simulink model "MdXXIsPosChk"  (R2024b)
settings: Solver=FixedStepDiscrete  StartTime=0.0  StopTime=10.0  FixedStep=0.01  RelTol=1e-3
libraries: simulink x35
(part 1 of 2)
settings Model: Creator=sn2xws  LastModifiedBy=sn55gm
settings Model: ModifiedHistory=|
  | 2024.5.6
  | 557 新增零重力电机
  | V3.0.1 2024.7.9 557模式流程V1.9
  | V3.0.2 2024.8.14 修复6slug无法报成功的问题
  | V3.0.3 Md18报成功的逻辑变更
  | V3.0.4 Md29报成功逻辑变更
  | V3.0.5 Md2，Md3，Md29到位置的逻辑更改（BUG924822）
  | V3.0.6 Md2，Md3，Md29到位置的逻辑更改（BUG924822），会默认到位置，需要先把到位置位置0
  | V3.0.7 Md32 只要靠背折叠到位置，modeposalready赋值1
  | V3.0.8 Md12 不看副驾到位
  | V3.0.9 Md30 Md31成功不看副驾前后
  | V3.1.0 Md30 Md31posalready 也不看副驾前后
  | V3.13.0 Md30 Md31成功不看二排腿托和延伸
settings SolverCC: AlgebraicLoopSolver=TrustRegion
settings DataIOCC: SaveFormat=StructureWithTime  ReturnWorkspaceOutputs=off
settings OptimizationCC: DefaultParameterBehavior=Inlined  EnhancedBackFolding=on  PassReuseOutputArgsAs=Individual arguments  ZeroExternalMemoryAtStartup=off  ZeroInternalMemoryAtStartup=off  OptimizeBlockOrder=speed  DifferentSizesBufferReuse=on  OptimizationCustomize=off  EfficientTunableParamExpr=on
settings DebuggingCC: ParameterTunabilityLossMsg=error  UnconnectedInputMsg=warning  UnconnectedOutputMsg=warning  UnconnectedLineMsg=warning  ArithmeticOperatorsInVariantConditions=warning
settings ModelReferenceCC: EnableRefExpFcnMdlSchedulingChecks=on  ModelReferenceNumInstancesAllowed=Single
settings SFSimCC: MATLABDynamicMemAlloc=off  CustomCodeUndefinedFunction=UseInterfaceOnly
settings RTWCC: Description=AUTOSAR  SystemTargetFile=autosar.tlc  GenCodeOnly=on  TemplateMakefile=ert_default_tmf  GenerateReport=on  IncludeHyperlinkInReport=on  LaunchReport=on  DataTypeReplacement=CDataTypesFixedWidth  GenerateTraceInfo=on  GenerateTraceReport=on  GenerateTraceReportSl=on  GenerateTraceReportSf=on  GenerateTraceReportEml=on  GenerateCodeMetricsReport=on  GPUComputeCapability=3.5
settings CodeAppCC: ForceParamTrailComments=on  IgnoreCustomStorageClasses=off  OperatorAnnotations=on  SimulinkDataObjDesc=on  SFDataObjDesc=on  InsertBlockDesc=on
settings STFCustomTargetCC: TargetLangStandard=C99 (ISO)  MultiwordLength=256  ParMdlRefBuildCompliant=on  CompOptLevelCompliant=on  IncludeMdlTerminateFcn=off  CombineOutputUpdateFcns=on  SuppressErrorStatus=on  ERTCustomFileBanners=on  SupportNonFinite=off  SupportComplex=off  SupportContinuousTime=off  SupportNonInlinedSFcns=off  RemoveResetFunc=on  MATLABClassNameForMDSCustomization=Simulink.SoftwareTarget.ERTCustomization  AutosarCompliant=on  UseToolchainInfoCompliant=on  LookupTableObjectStructAxisOrder=2,1,3,4,...  LUTObjectStructOrderEvenSpacing=Size,Table,Breakpoints  SystemTargetFile=autosar.tlc
settings ERTTargetCC: TargetLangStandard=C99 (ISO)  ConcurrentExecutionCompliant=off  IncludeMdlTerminateFcn=off  SuppressErrorStatus=on  SupportNonFinite=off  SupportComplex=off  ModelStepFunctionPrototypeControlCompliant=off  CPPClassGenCompliant=off  AutosarCompliant=on  LookupTableObjectStructAxisOrder=2,1,3,4,...  LUTObjectStructOrderEvenSpacing=Size,Table,Breakpoints  ERTCustomFileTemplate=example_file_process.tlc  ERTFilePackagingFormat=Compact  BooleanTrueId=TRUE  BooleanFalseId=FALSE  DynamicArrayContainerType=coder::array

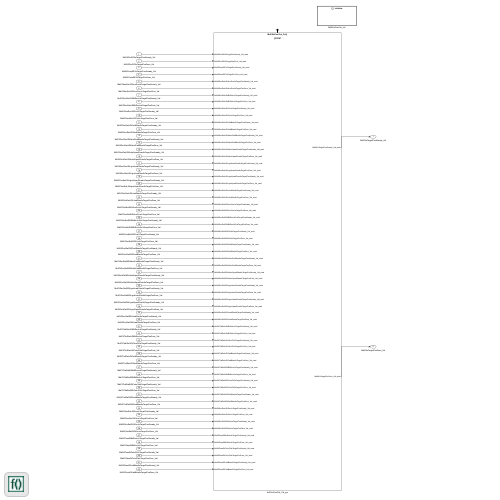
[thumbnail: Simulink's stored preview of the top-level diagram]
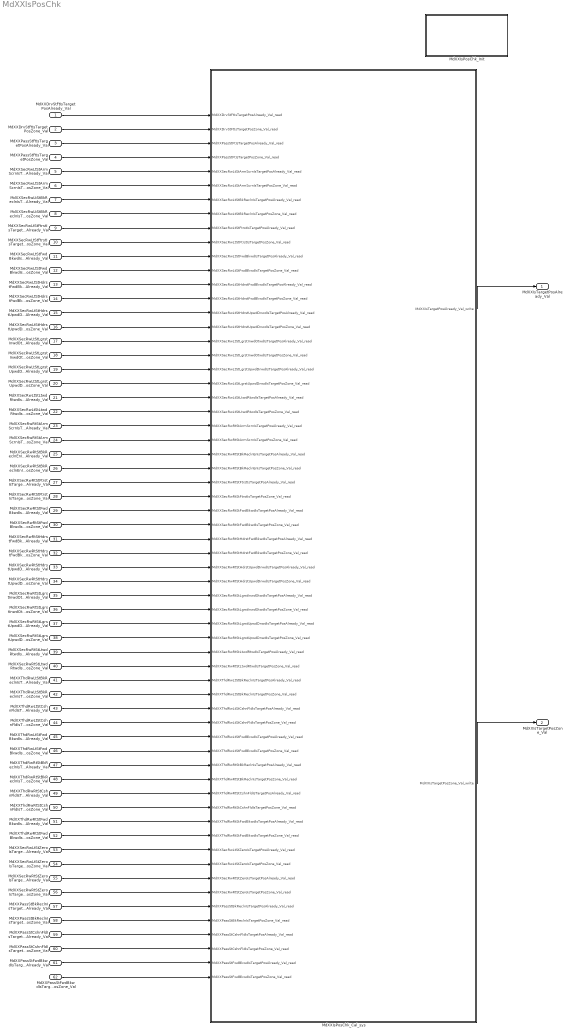
== system MdXXIsPosChk ==
  MdXXDrvStFtIsTargetPosAlready_Val : Inport  OutDataTypeStr=uint32  PortDimensions=1
  MdXXDrvStFtIsTargetPosZone_Val : Inport  Port=2  OutDataTypeStr=uint32  PortDimensions=1
  MdXXPassStFtIsTargetPosAlready_Val : Inport  Port=3  OutDataTypeStr=uint32  PortDimensions=1
  MdXXPassStFtIsTargetPosZone_Val : Inport  Port=4  OutDataTypeStr=uint32  PortDimensions=1
  MdXXSecRwLtStArmScrnIsTargetPosAlready_Val : Inport  Port=5  OutDataTypeStr=uint32  PortDimensions=1
  MdXXSecRwLtStArmScrnIsTargetPosZone_Val : Inport  Port=6  OutDataTypeStr=uint32  PortDimensions=1
  MdXXSecRwLtStBkReclnIsTargetPosAlready_Val : Inport  Port=7  OutDataTypeStr=uint32  PortDimensions=1
  MdXXSecRwLtStBkReclnIsTargetPosZone_Val : Inport  Port=8  OutDataTypeStr=uint32  PortDimensions=1
  MdXXSecRwLtStFtrstIsTargetPosAlready_Val : Inport  Port=9  OutDataTypeStr=uint32  PortDimensions=1
  MdXXSecRwLtStFtrstIsTargetPosZone_Val : Inport  Port=10  OutDataTypeStr=uint32  PortDimensions=1
  MdXXSecRwLtStFwdBkwdIsTargetPosAlready_Val : Inport  Port=11  OutDataTypeStr=uint32  PortDimensions=1
  MdXXSecRwLtStFwdBkwdIsTargetPosZone_Val : Inport  Port=12  OutDataTypeStr=uint32  PortDimensions=1
  MdXXSecRwLtStHdrstFwdBkwdIsTargetPosAlready_Val : Inport  Port=13  OutDataTypeStr=uint32  PortDimensions=1
  MdXXSecRwLtStHdrstFwdBkwdIsTargetPosZone_Val : Inport  Port=14  OutDataTypeStr=uint32  PortDimensions=1
  MdXXSecRwLtStHdrstUpwdDnwdIsTargetPosAlready_Val : Inport  Port=15  OutDataTypeStr=uint32  PortDimensions=1
  MdXXSecRwLtStHdrstUpwdDnwdIsTargetPosZone_Val : Inport  Port=16  OutDataTypeStr=uint32  PortDimensions=1
  MdXXSecRwLtStLgrstInwdOtwdIsTargetPosAlready_Val : Inport  Port=17  OutDataTypeStr=uint32  PortDimensions=1
  MdXXSecRwLtStLgrstInwdOtwdIsTargetPosZone_Val : Inport  Port=18  OutDataTypeStr=uint32  PortDimensions=1
  MdXXSecRwLtStLgrstUpwdDnwdIsTargetPosAlready_Val : Inport  Port=19  OutDataTypeStr=uint32  PortDimensions=1
  MdXXSecRwLtStLgrstUpwdDnwdIsTargetPosZone_Val : Inport  Port=20  OutDataTypeStr=uint32  PortDimensions=1
  MdXXSecRwLtStLtwdRtwdIsTargetPosAlready_Val : Inport  Port=21  OutDataTypeStr=uint32  PortDimensions=1
  MdXXSecRwLtStLtwdRtwdIsTargetPosZone_Val : Inport  Port=22  OutDataTypeStr=uint32  PortDimensions=1
  MdXXSecRwRtStArmScrnIsTargetPosAlready_Val : Inport  Port=23  OutDataTypeStr=uint32  PortDimensions=1
  MdXXSecRwRtStArmScrnIsTargetPosZone_Val : Inport  Port=24  OutDataTypeStr=uint32  PortDimensions=1
  MdXXSecRwRtStBkReclnEnIsTargetPosAlready_Val : Inport  Port=25  OutDataTypeStr=uint32  PortDimensions=1
  MdXXSecRwRtStBkReclnEnIsTargetPosZone_Val : Inport  Port=26  OutDataTypeStr=uint32  PortDimensions=1
  MdXXSecRwRtStFtrstIsTargetPosAlready_Val : Inport  Port=27  OutDataTypeStr=uint32  PortDimensions=1
  MdXXSecRwRtStFtrstIsTargetPosZone_Val : Inport  Port=28  OutDataTypeStr=uint32  PortDimensions=1
  MdXXSecRwRtStFwdBkwdIsTargetPosAlready_Val : Inport  Port=29  OutDataTypeStr=uint32  PortDimensions=1
  MdXXSecRwRtStFwdBkwdIsTargetPosZone_Val : Inport  Port=30  OutDataTypeStr=uint32  PortDimensions=1
  MdXXSecRwRtStHdrstFwdBkwdIsTargetPosAlready_Val : Inport  Port=31  OutDataTypeStr=uint32  PortDimensions=1
  MdXXSecRwRtStHdrstFwdBkwdIsTargetPosZone_Val : Inport  Port=32  OutDataTypeStr=uint32  PortDimensions=1
  MdXXSecRwRtStHdrstUpwdDnwdIsTargetPosAlready_Val : Inport  Port=33  OutDataTypeStr=uint32  PortDimensions=1
  MdXXSecRwRtStHdrstUpwdDnwdIsTargetPosZone_Val : Inport  Port=34  OutDataTypeStr=uint32  PortDimensions=1
  MdXXSecRwRtStLgrstInwdOtwdIsTargetPosAlready_Val : Inport  Port=35  OutDataTypeStr=uint32  PortDimensions=1
  MdXXSecRwRtStLgrstInwdOtwdIsTargetPosZone_Val : Inport  Port=36  OutDataTypeStr=uint32  PortDimensions=1
  MdXXSecRwRtStLgrstUpwdDnwdIsTargetPosAlready_Val : Inport  Port=37  OutDataTypeStr=uint32  PortDimensions=1
  MdXXSecRwRtStLgrstUpwdDnwdIsTargetPosZone_Val : Inport  Port=38  OutDataTypeStr=uint32  PortDimensions=1
  MdXXSecRwRtStLtwdRtwdIsTargetPosAlready_Val : Inport  Port=39  OutDataTypeStr=uint32  PortDimensions=1
  MdXXSecRwRtStLtwdRtwdIsTargetPosZone_Val : Inport  Port=40  OutDataTypeStr=uint32  PortDimensions=1
  MdXXThdRwLtStBkReclnIsTargetPosAlready_Val : Inport  Port=41  OutDataTypeStr=uint32  PortDimensions=1
  MdXXThdRwLtStBkReclnIsTargetPosZone_Val : Inport  Port=42  OutDataTypeStr=uint32  PortDimensions=1
  MdXXThdRwLtStCshnFldIsTargetPosAlready_Val : Inport  Port=43  OutDataTypeStr=uint32  PortDimensions=1
  MdXXThdRwLtStCshnFldIsTargetPosZone_Val : Inport  Port=44  OutDataTypeStr=uint32  PortDimensions=1
  MdXXThdRwLtStFwdBkwdIsTargetPosAlready_Val : Inport  Port=45  OutDataTypeStr=uint32  PortDimensions=1
  MdXXThdRwLtStFwdBkwdIsTargetPosZone_Val : Inport  Port=46  OutDataTypeStr=uint32  PortDimensions=1
  MdXXThdRwRtStBkReclnIsTargetPosAlready_Val : Inport  Port=47  OutDataTypeStr=uint32  PortDimensions=1
  MdXXThdRwRtStBkReclnIsTargetPosZone_Val : Inport  Port=48  OutDataTypeStr=uint32  PortDimensions=1
  MdXXThdRwRtStCshnFldIsTargetPosAlready_Val : Inport  Port=49  OutDataTypeStr=uint32  PortDimensions=1
  MdXXThdRwRtStCshnFldIsTargetPosZone_Val : Inport  Port=50  OutDataTypeStr=uint32  PortDimensions=1
  MdXXThdRwRtStFwdBkwdIsTargetPosAlready_Val : Inport  Port=51  OutDataTypeStr=uint32  PortDimensions=1
  MdXXThdRwRtStFwdBkwdIsTargetPosZone_Val : Inport  Port=52  OutDataTypeStr=uint32  PortDimensions=1
  MdXXSecRwLtStZeroIsTargetPosAlready_Val : Inport  Port=53  OutDataTypeStr=uint32  PortDimensions=1
  MdXXSecRwLtStZeroIsTargetPosZone_Val : Inport  Port=54  OutDataTypeStr=uint32  PortDimensions=1
  MdXXSecRwRtStZeroIsTargetPosAlready_Val : Inport  Port=55  OutDataTypeStr=uint32  PortDimensions=1
  MdXXSecRwRtStZeroIsTargetPosZone_Val : Inport  Port=56  OutDataTypeStr=uint32  PortDimensions=1
  MdXXPassStBkReclnIsTargetPosAlready_Val : Inport  Port=57  OutDataTypeStr=uint32  PortDimensions=1
  MdXXPassStBkReclnIsTargetPosZone_Val : Inport  Port=58  OutDataTypeStr=uint32  PortDimensions=1
  MdXXPassStCshnFldIsTargetPosAlready_Val : Inport  Port=59  OutDataTypeStr=uint32  PortDimensions=1
  MdXXPassStCshnFldIsTargetPosZone_Val : Inport  Port=60  OutDataTypeStr=uint32  PortDimensions=1
  MdXXPassStFwdBkwdIsTargetPosAlready_Val : Inport  Port=61  OutDataTypeStr=uint32  PortDimensions=1
  MdXXPassStFwdBkwdIsTargetPosZone_Val : Inport  Port=62  OutDataTypeStr=uint32  PortDimensions=1
  MdXXIsPosChk_Cal_sys : Subsystem
  MdXXIsPosChk_Init : Subsystem
  MdXXIsTargetPosAlready_Val : Outport  OutDataTypeStr=uint32  PortDimensions=1  VectorParamsAs1DForOutWhenUnconnected=off
  MdXXIsTargetPosZone_Val : Outport  Port=2  OutDataTypeStr=uint32  PortDimensions=1  VectorParamsAs1DForOutWhenUnconnected=off
  wires:
  MdXXDrvStFtIsTargetPosAlready_Val/1 -> MdXXIsPosChk_Cal_sys/1(MdXXDrvStFtIsTargetPosAlready_Val_read)
  MdXXDrvStFtIsTargetPosZone_Val/1 -> MdXXIsPosChk_Cal_sys/2(MdXXDrvStFtIsTargetPosZone_Val_read)
  MdXXPassStFtIsTargetPosAlready_Val/1 -> MdXXIsPosChk_Cal_sys/3(MdXXPassStFtIsTargetPosAlready_Val_read)
  MdXXPassStFtIsTargetPosZone_Val/1 -> MdXXIsPosChk_Cal_sys/4(MdXXPassStFtIsTargetPosZone_Val_read)
  MdXXSecRwLtStArmScrnIsTargetPosAlready_Val/1 -> MdXXIsPosChk_Cal_sys/5(MdXXSecRwLtStArmScrnIsTargetPosAlready_Val_read)
  MdXXSecRwLtStArmScrnIsTargetPosZone_Val/1 -> MdXXIsPosChk_Cal_sys/6(MdXXSecRwLtStArmScrnIsTargetPosZone_Val_read)
  MdXXSecRwLtStBkReclnIsTargetPosAlready_Val/1 -> MdXXIsPosChk_Cal_sys/7(MdXXSecRwLtStBkReclnIsTargetPosAlready_Val_read)
  MdXXSecRwLtStBkReclnIsTargetPosZone_Val/1 -> MdXXIsPosChk_Cal_sys/8(MdXXSecRwLtStBkReclnIsTargetPosZone_Val_read)
  MdXXSecRwLtStFtrstIsTargetPosAlready_Val/1 -> MdXXIsPosChk_Cal_sys/9(MdXXSecRwLtStFtrstIsTargetPosAlready_Val_read)
  MdXXSecRwLtStFtrstIsTargetPosZone_Val/1 -> MdXXIsPosChk_Cal_sys/10(MdXXSecRwLtStFtrstIsTargetPosZone_Val_read)
  MdXXSecRwLtStFwdBkwdIsTargetPosAlready_Val/1 -> MdXXIsPosChk_Cal_sys/11(MdXXSecRwLtStFwdBkwdIsTargetPosAlready_Val_read)
  MdXXSecRwLtStFwdBkwdIsTargetPosZone_Val/1 -> MdXXIsPosChk_Cal_sys/12(MdXXSecRwLtStFwdBkwdIsTargetPosZone_Val_read)
  MdXXSecRwLtStHdrstFwdBkwdIsTargetPosAlready_Val/1 -> MdXXIsPosChk_Cal_sys/13(MdXXSecRwLtStHdrstFwdBkwdIsTargetPosAlready_Val_read)
  MdXXSecRwLtStHdrstFwdBkwdIsTargetPosZone_Val/1 -> MdXXIsPosChk_Cal_sys/14(MdXXSecRwLtStHdrstFwdBkwdIsTargetPosZone_Val_read)
  MdXXSecRwLtStHdrstUpwdDnwdIsTargetPosAlready_Val/1 -> MdXXIsPosChk_Cal_sys/15(MdXXSecRwLtStHdrstUpwdDnwdIsTargetPosAlready_Val_read)
  MdXXSecRwLtStHdrstUpwdDnwdIsTargetPosZone_Val/1 -> MdXXIsPosChk_Cal_sys/16(MdXXSecRwLtStHdrstUpwdDnwdIsTargetPosZone_Val_read)
  MdXXSecRwLtStLgrstInwdOtwdIsTargetPosAlready_Val/1 -> MdXXIsPosChk_Cal_sys/17(MdXXSecRwLtStLgrstInwdOtwdIsTargetPosAlready_Val_read)
  MdXXSecRwLtStLgrstInwdOtwdIsTargetPosZone_Val/1 -> MdXXIsPosChk_Cal_sys/18(MdXXSecRwLtStLgrstInwdOtwdIsTargetPosZone_Val_read)
  MdXXSecRwLtStLgrstUpwdDnwdIsTargetPosAlready_Val/1 -> MdXXIsPosChk_Cal_sys/19(MdXXSecRwLtStLgrstUpwdDnwdIsTargetPosAlready_Val_read)
  MdXXSecRwLtStLgrstUpwdDnwdIsTargetPosZone_Val/1 -> MdXXIsPosChk_Cal_sys/20(MdXXSecRwLtStLgrstUpwdDnwdIsTargetPosZone_Val_read)
  MdXXSecRwLtStLtwdRtwdIsTargetPosAlready_Val/1 -> MdXXIsPosChk_Cal_sys/21(MdXXSecRwLtStLtwdRtwdIsTargetPosAlready_Val_read)
  MdXXSecRwLtStLtwdRtwdIsTargetPosZone_Val/1 -> MdXXIsPosChk_Cal_sys/22(MdXXSecRwLtStLtwdRtwdIsTargetPosZone_Val_read)
  MdXXSecRwRtStArmScrnIsTargetPosAlready_Val/1 -> MdXXIsPosChk_Cal_sys/23(MdXXSecRwRtStArmScrnIsTargetPosAlready_Val_read)
  MdXXSecRwRtStArmScrnIsTargetPosZone_Val/1 -> MdXXIsPosChk_Cal_sys/24(MdXXSecRwRtStArmScrnIsTargetPosZone_Val_read)
  MdXXSecRwRtStBkReclnEnIsTargetPosAlready_Val/1 -> MdXXIsPosChk_Cal_sys/25(MdXXSecRwRtStBkReclnEnIsTargetPosAlready_Val_read)
  MdXXSecRwRtStBkReclnEnIsTargetPosZone_Val/1 -> MdXXIsPosChk_Cal_sys/26(MdXXSecRwRtStBkReclnEnIsTargetPosZone_Val_read)
  MdXXSecRwRtStFtrstIsTargetPosAlready_Val/1 -> MdXXIsPosChk_Cal_sys/27(MdXXSecRwRtStFtrstIsTargetPosAlready_Val_read)
  MdXXSecRwRtStFtrstIsTargetPosZone_Val/1 -> MdXXIsPosChk_Cal_sys/28(MdXXSecRwRtStFtrstIsTargetPosZone_Val_read)
  MdXXSecRwRtStFwdBkwdIsTargetPosAlready_Val/1 -> MdXXIsPosChk_Cal_sys/29(MdXXSecRwRtStFwdBkwdIsTargetPosAlready_Val_read)
  MdXXSecRwRtStFwdBkwdIsTargetPosZone_Val/1 -> MdXXIsPosChk_Cal_sys/30(MdXXSecRwRtStFwdBkwdIsTargetPosZone_Val_read)
  MdXXSecRwRtStHdrstFwdBkwdIsTargetPosAlready_Val/1 -> MdXXIsPosChk_Cal_sys/31(MdXXSecRwRtStHdrstFwdBkwdIsTargetPosAlready_Val_read)
  MdXXSecRwRtStHdrstFwdBkwdIsTargetPosZone_Val/1 -> MdXXIsPosChk_Cal_sys/32(MdXXSecRwRtStHdrstFwdBkwdIsTargetPosZone_Val_read)
  MdXXSecRwRtStHdrstUpwdDnwdIsTargetPosAlready_Val/1 -> MdXXIsPosChk_Cal_sys/33(MdXXSecRwRtStHdrstUpwdDnwdIsTargetPosAlready_Val_read)
  MdXXSecRwRtStHdrstUpwdDnwdIsTargetPosZone_Val/1 -> MdXXIsPosChk_Cal_sys/34(MdXXSecRwRtStHdrstUpwdDnwdIsTargetPosZone_Val_read)
  MdXXSecRwRtStLgrstInwdOtwdIsTargetPosAlready_Val/1 -> MdXXIsPosChk_Cal_sys/35(MdXXSecRwRtStLgrstInwdOtwdIsTargetPosAlready_Val_read)
  MdXXSecRwRtStLgrstInwdOtwdIsTargetPosZone_Val/1 -> MdXXIsPosChk_Cal_sys/36(MdXXSecRwRtStLgrstInwdOtwdIsTargetPosZone_Val_read)
  MdXXSecRwRtStLgrstUpwdDnwdIsTargetPosAlready_Val/1 -> MdXXIsPosChk_Cal_sys/37(MdXXSecRwRtStLgrstUpwdDnwdIsTargetPosAlready_Val_read)
  MdXXSecRwRtStLgrstUpwdDnwdIsTargetPosZone_Val/1 -> MdXXIsPosChk_Cal_sys/38(MdXXSecRwRtStLgrstUpwdDnwdIsTargetPosZone_Val_read)
  MdXXSecRwRtStLtwdRtwdIsTargetPosAlready_Val/1 -> MdXXIsPosChk_Cal_sys/39(MdXXSecRwRtStLtwdRtwdIsTargetPosAlready_Val_read)
  MdXXSecRwRtStLtwdRtwdIsTargetPosZone_Val/1 -> MdXXIsPosChk_Cal_sys/40(MdXXSecRwRtStLtwdRtwdIsTargetPosZone_Val_read)
  MdXXThdRwLtStBkReclnIsTargetPosAlready_Val/1 -> MdXXIsPosChk_Cal_sys/41(MdXXThdRwLtStBkReclnIsTargetPosAlready_Val_read)
  MdXXThdRwLtStBkReclnIsTargetPosZone_Val/1 -> MdXXIsPosChk_Cal_sys/42(MdXXThdRwLtStBkReclnIsTargetPosZone_Val_read)
  MdXXThdRwLtStCshnFldIsTargetPosAlready_Val/1 -> MdXXIsPosChk_Cal_sys/43(MdXXThdRwLtStCshnFldIsTargetPosAlready_Val_read)
  MdXXThdRwLtStCshnFldIsTargetPosZone_Val/1 -> MdXXIsPosChk_Cal_sys/44(MdXXThdRwLtStCshnFldIsTargetPosZone_Val_read)
  MdXXThdRwLtStFwdBkwdIsTargetPosAlready_Val/1 -> MdXXIsPosChk_Cal_sys/45(MdXXThdRwLtStFwdBkwdIsTargetPosAlready_Val_read)
  MdXXThdRwLtStFwdBkwdIsTargetPosZone_Val/1 -> MdXXIsPosChk_Cal_sys/46(MdXXThdRwLtStFwdBkwdIsTargetPosZone_Val_read)
  MdXXThdRwRtStBkReclnIsTargetPosAlready_Val/1 -> MdXXIsPosChk_Cal_sys/47(MdXXThdRwRtStBkReclnIsTargetPosAlready_Val_read)
  MdXXThdRwRtStBkReclnIsTargetPosZone_Val/1 -> MdXXIsPosChk_Cal_sys/48(MdXXThdRwRtStBkReclnIsTargetPosZone_Val_read)
  MdXXThdRwRtStCshnFldIsTargetPosAlready_Val/1 -> MdXXIsPosChk_Cal_sys/49(MdXXThdRwRtStCshnFldIsTargetPosAlready_Val_read)
  MdXXThdRwRtStCshnFldIsTargetPosZone_Val/1 -> MdXXIsPosChk_Cal_sys/50(MdXXThdRwRtStCshnFldIsTargetPosZone_Val_read)
  MdXXThdRwRtStFwdBkwdIsTargetPosAlready_Val/1 -> MdXXIsPosChk_Cal_sys/51(MdXXThdRwRtStFwdBkwdIsTargetPosAlready_Val_read)
  MdXXThdRwRtStFwdBkwdIsTargetPosZone_Val/1 -> MdXXIsPosChk_Cal_sys/52(MdXXThdRwRtStFwdBkwdIsTargetPosZone_Val_read)
  MdXXIsPosChk_Cal_sys/1(MdXXIsTargetPosAlready_Val_write) -> MdXXIsTargetPosAlready_Val/1
  MdXXIsPosChk_Cal_sys/2(MdXXIsTargetPosZone_Val_write) -> MdXXIsTargetPosZone_Val/1
  MdXXSecRwLtStZeroIsTargetPosAlready_Val/1 -> MdXXIsPosChk_Cal_sys/53(MdXXSecRwLtStZeroIsTargetPosAlready_Val_read)
  MdXXSecRwLtStZeroIsTargetPosZone_Val/1 -> MdXXIsPosChk_Cal_sys/54(MdXXSecRwLtStZeroIsTargetPosZone_Val_read)
  MdXXSecRwRtStZeroIsTargetPosAlready_Val/1 -> MdXXIsPosChk_Cal_sys/55(MdXXSecRwRtStZeroIsTargetPosAlready_Val_read)
  MdXXSecRwRtStZeroIsTargetPosZone_Val/1 -> MdXXIsPosChk_Cal_sys/56(MdXXSecRwRtStZeroIsTargetPosZone_Val_read)
  MdXXPassStBkReclnIsTargetPosAlready_Val/1 -> MdXXIsPosChk_Cal_sys/57(MdXXPassStBkReclnIsTargetPosAlready_Val_read)
  MdXXPassStBkReclnIsTargetPosZone_Val/1 -> MdXXIsPosChk_Cal_sys/58(MdXXPassStBkReclnIsTargetPosZone_Val_read)
  MdXXPassStCshnFldIsTargetPosAlready_Val/1 -> MdXXIsPosChk_Cal_sys/59(MdXXPassStCshnFldIsTargetPosAlready_Val_read)
  MdXXPassStCshnFldIsTargetPosZone_Val/1 -> MdXXIsPosChk_Cal_sys/60(MdXXPassStCshnFldIsTargetPosZone_Val_read)
  MdXXPassStFwdBkwdIsTargetPosAlready_Val/1 -> MdXXIsPosChk_Cal_sys/61(MdXXPassStFwdBkwdIsTargetPosAlready_Val_read)
  MdXXPassStFwdBkwdIsTargetPosZone_Val/1 -> MdXXIsPosChk_Cal_sys/62(MdXXPassStFwdBkwdIsTargetPosZone_Val_read)

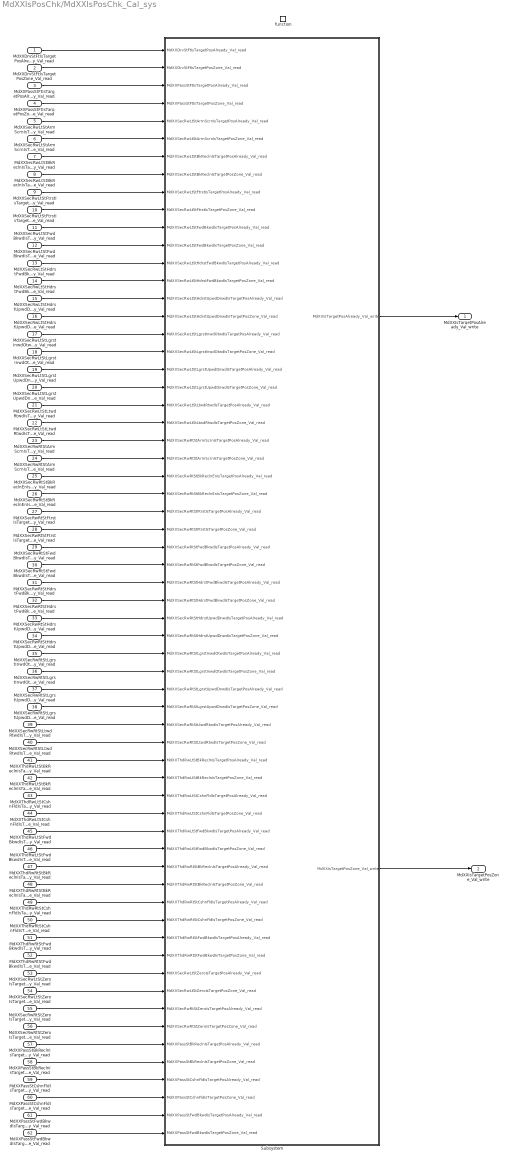
== system MdXXIsPosChk/MdXXIsPosChk_Cal_sys ==
  MdXXDrvStFtIsTargetPosAlready_Val_read : Inport
  MdXXDrvStFtIsTargetPosZone_Val_read : Inport  Port=2
  MdXXPassStFtIsTargetPosAlready_Val_read : Inport  Port=3
  MdXXPassStFtIsTargetPosZone_Val_read : Inport  Port=4
  MdXXSecRwLtStArmScrnIsTargetPosAlready_Val_read : Inport  Port=5
  MdXXSecRwLtStArmScrnIsTargetPosZone_Val_read : Inport  Port=6
  MdXXSecRwLtStBkReclnIsTargetPosAlready_Val_read : Inport  Port=7
  MdXXSecRwLtStBkReclnIsTargetPosZone_Val_read : Inport  Port=8
  MdXXSecRwLtStFtrstIsTargetPosAlready_Val_read : Inport  Port=9
  MdXXSecRwLtStFtrstIsTargetPosZone_Val_read : Inport  Port=10
  MdXXSecRwLtStFwdBkwdIsTargetPosAlready_Val_read : Inport  Port=11
  MdXXSecRwLtStFwdBkwdIsTargetPosZone_Val_read : Inport  Port=12
  MdXXSecRwLtStHdrstFwdBkwdIsTargetPosAlready_Val_read : Inport  Port=13
  MdXXSecRwLtStHdrstFwdBkwdIsTargetPosZone_Val_read : Inport  Port=14
  MdXXSecRwLtStHdrstUpwdDnwdIsTargetPosAlready_Val_read : Inport  Port=15
  MdXXSecRwLtStHdrstUpwdDnwdIsTargetPosZone_Val_read : Inport  Port=16
  MdXXSecRwLtStLgrstInwdOtwdIsTargetPosAlready_Val_read : Inport  Port=17
  MdXXSecRwLtStLgrstInwdOtwdIsTargetPosZone_Val_read : Inport  Port=18
  MdXXSecRwLtStLgrstUpwdDnwdIsTargetPosAlready_Val_read : Inport  Port=19
  MdXXSecRwLtStLgrstUpwdDnwdIsTargetPosZone_Val_read : Inport  Port=20
  MdXXSecRwLtStLtwdRtwdIsTargetPosAlready_Val_read : Inport  Port=21
  MdXXSecRwLtStLtwdRtwdIsTargetPosZone_Val_read : Inport  Port=22
  MdXXSecRwRtStArmScrnIsTargetPosAlready_Val_read : Inport  Port=23
  MdXXSecRwRtStArmScrnIsTargetPosZone_Val_read : Inport  Port=24
  MdXXSecRwRtStBkReclnEnIsTargetPosAlready_Val_read : Inport  Port=25
  MdXXSecRwRtStBkReclnEnIsTargetPosZone_Val_read : Inport  Port=26
  MdXXSecRwRtStFtrstIsTargetPosAlready_Val_read : Inport  Port=27
  MdXXSecRwRtStFtrstIsTargetPosZone_Val_read : Inport  Port=28
  MdXXSecRwRtStFwdBkwdIsTargetPosAlready_Val_read : Inport  Port=29
  MdXXSecRwRtStFwdBkwdIsTargetPosZone_Val_read : Inport  Port=30
  MdXXSecRwRtStHdrstFwdBkwdIsTargetPosAlready_Val_read : Inport  Port=31
  MdXXSecRwRtStHdrstFwdBkwdIsTargetPosZone_Val_read : Inport  Port=32
  MdXXSecRwRtStHdrstUpwdDnwdIsTargetPosAlready_Val_read : Inport  Port=33
  MdXXSecRwRtStHdrstUpwdDnwdIsTargetPosZone_Val_read : Inport  Port=34
  MdXXSecRwRtStLgrstInwdOtwdIsTargetPosAlready_Val_read : Inport  Port=35
  MdXXSecRwRtStLgrstInwdOtwdIsTargetPosZone_Val_read : Inport  Port=36
  MdXXSecRwRtStLgrstUpwdDnwdIsTargetPosAlready_Val_read : Inport  Port=37
  MdXXSecRwRtStLgrstUpwdDnwdIsTargetPosZone_Val_read : Inport  Port=38
  MdXXSecRwRtStLtwdRtwdIsTargetPosAlready_Val_read : Inport  Port=39
  MdXXSecRwRtStLtwdRtwdIsTargetPosZone_Val_read : Inport  Port=40
  MdXXThdRwLtStBkReclnIsTargetPosAlready_Val_read : Inport  Port=41
  MdXXThdRwLtStBkReclnIsTargetPosZone_Val_read : Inport  Port=42
  MdXXThdRwLtStCshnFldIsTargetPosAlready_Val_read : Inport  Port=43
  MdXXThdRwLtStCshnFldIsTargetPosZone_Val_read : Inport  Port=44
  MdXXThdRwLtStFwdBkwdIsTargetPosAlready_Val_read : Inport  Port=45
  MdXXThdRwLtStFwdBkwdIsTargetPosZone_Val_read : Inport  Port=46
  MdXXThdRwRtStBkReclnIsTargetPosAlready_Val_read : Inport  Port=47
  MdXXThdRwRtStBkReclnIsTargetPosZone_Val_read : Inport  Port=48
  MdXXThdRwRtStCshnFldIsTargetPosAlready_Val_read : Inport  Port=49
  MdXXThdRwRtStCshnFldIsTargetPosZone_Val_read : Inport  Port=50
  MdXXThdRwRtStFwdBkwdIsTargetPosAlready_Val_read : Inport  Port=51
  MdXXThdRwRtStFwdBkwdIsTargetPosZone_Val_read : Inport  Port=52
  MdXXSecRwLtStZeroIsTargetPosAlready_Val_read : Inport  Port=53
  MdXXSecRwLtStZeroIsTargetPosZone_Val_read : Inport  Port=54
  MdXXSecRwRtStZeroIsTargetPosAlready_Val_read : Inport  Port=55
  MdXXSecRwRtStZeroIsTargetPosZone_Val_read : Inport  Port=56
  MdXXPassStBkReclnIsTargetPosAlready_Val_read : Inport  Port=57
  MdXXPassStBkReclnIsTargetPosZone_Val_read : Inport  Port=58
  MdXXPassStCshnFldIsTargetPosAlready_Val_read : Inport  Port=59
  MdXXPassStCshnFldIsTargetPosZone_Val_read : Inport  Port=60
  MdXXPassStFwdBkwdIsTargetPosAlready_Val_read : Inport  Port=61
  MdXXPassStFwdBkwdIsTargetPosZone_Val_read : Inport  Port=62
  function : TriggerPort  TriggerType=function-call  IsSimulinkFunction=on  FunctionName=MdXXIsPosChk_Cal  VariantControl=(inherit)
  Subsystem : Subsystem
  MdXXIsTargetPosAlready_Val_write : Outport  VectorParamsAs1DForOutWhenUnconnected=off
      settings: EnsureOutportIsVirtual=on
  MdXXIsTargetPosZone_Val_write : Outport  Port=2  VectorParamsAs1DForOutWhenUnconnected=off
      settings: EnsureOutportIsVirtual=on
  wires:
  MdXXSecRwLtStArmScrnIsTargetPosZone_Val_read/1 -> Subsystem/6(MdXXSecRwLtStArmScrnIsTargetPosZone_Val_read)
  MdXXSecRwLtStBkReclnIsTargetPosAlready_Val_read/1 -> Subsystem/7(MdXXSecRwLtStBkReclnIsTargetPosAlready_Val_read)
  MdXXSecRwLtStBkReclnIsTargetPosZone_Val_read/1 -> Subsystem/8(MdXXSecRwLtStBkReclnIsTargetPosZone_Val_read)
  MdXXPassStFtIsTargetPosZone_Val_read/1 -> Subsystem/4(MdXXPassStFtIsTargetPosZone_Val_read)
  MdXXSecRwLtStArmScrnIsTargetPosAlready_Val_read/1 -> Subsystem/5(MdXXSecRwLtStArmScrnIsTargetPosAlready_Val_read)
  MdXXSecRwLtStFtrstIsTargetPosAlready_Val_read/1 -> Subsystem/9(MdXXSecRwLtStFtrstIsTargetPosAlready_Val_read)
  MdXXSecRwLtStFtrstIsTargetPosZone_Val_read/1 -> Subsystem/10(MdXXSecRwLtStFtrstIsTargetPosZone_Val_read)
  MdXXDrvStFtIsTargetPosAlready_Val_read/1 -> Subsystem/1(MdXXDrvStFtIsTargetPosAlready_Val_read)
  MdXXDrvStFtIsTargetPosZone_Val_read/1 -> Subsystem/2(MdXXDrvStFtIsTargetPosZone_Val_read)
  MdXXPassStFtIsTargetPosAlready_Val_read/1 -> Subsystem/3(MdXXPassStFtIsTargetPosAlready_Val_read)
  MdXXSecRwLtStFwdBkwdIsTargetPosAlready_Val_read/1 -> Subsystem/11(MdXXSecRwLtStFwdBkwdIsTargetPosAlready_Val_read)
  MdXXSecRwLtStFwdBkwdIsTargetPosZone_Val_read/1 -> Subsystem/12(MdXXSecRwLtStFwdBkwdIsTargetPosZone_Val_read)
  MdXXSecRwLtStHdrstFwdBkwdIsTargetPosAlready_Val_read/1 -> Subsystem/13(MdXXSecRwLtStHdrstFwdBkwdIsTargetPosAlready_Val_read)
  MdXXSecRwLtStHdrstFwdBkwdIsTargetPosZone_Val_read/1 -> Subsystem/14(MdXXSecRwLtStHdrstFwdBkwdIsTargetPosZone_Val_read)
  MdXXSecRwLtStHdrstUpwdDnwdIsTargetPosAlready_Val_read/1 -> Subsystem/15(MdXXSecRwLtStHdrstUpwdDnwdIsTargetPosAlready_Val_read)
  MdXXSecRwLtStHdrstUpwdDnwdIsTargetPosZone_Val_read/1 -> Subsystem/16(MdXXSecRwLtStHdrstUpwdDnwdIsTargetPosZone_Val_read)
  MdXXSecRwLtStLgrstInwdOtwdIsTargetPosAlready_Val_read/1 -> Subsystem/17(MdXXSecRwLtStLgrstInwdOtwdIsTargetPosAlready_Val_read)
  MdXXSecRwLtStLgrstInwdOtwdIsTargetPosZone_Val_read/1 -> Subsystem/18(MdXXSecRwLtStLgrstInwdOtwdIsTargetPosZone_Val_read)
  MdXXSecRwLtStLgrstUpwdDnwdIsTargetPosAlready_Val_read/1 -> Subsystem/19(MdXXSecRwLtStLgrstUpwdDnwdIsTargetPosAlready_Val_read)
  MdXXSecRwLtStLgrstUpwdDnwdIsTargetPosZone_Val_read/1 -> Subsystem/20(MdXXSecRwLtStLgrstUpwdDnwdIsTargetPosZone_Val_read)
  MdXXSecRwLtStLtwdRtwdIsTargetPosAlready_Val_read/1 -> Subsystem/21(MdXXSecRwLtStLtwdRtwdIsTargetPosAlready_Val_read)
  MdXXSecRwLtStLtwdRtwdIsTargetPosZone_Val_read/1 -> Subsystem/22(MdXXSecRwLtStLtwdRtwdIsTargetPosZone_Val_read)
  MdXXSecRwRtStArmScrnIsTargetPosAlready_Val_read/1 -> Subsystem/23(MdXXSecRwRtStArmScrnIsTargetPosAlready_Val_read)
  MdXXSecRwRtStArmScrnIsTargetPosZone_Val_read/1 -> Subsystem/24(MdXXSecRwRtStArmScrnIsTargetPosZone_Val_read)
  MdXXSecRwRtStBkReclnEnIsTargetPosAlready_Val_read/1 -> Subsystem/25(MdXXSecRwRtStBkReclnEnIsTargetPosAlready_Val_read)
  MdXXSecRwRtStBkReclnEnIsTargetPosZone_Val_read/1 -> Subsystem/26(MdXXSecRwRtStBkReclnEnIsTargetPosZone_Val_read)
  MdXXSecRwRtStFtrstIsTargetPosAlready_Val_read/1 -> Subsystem/27(MdXXSecRwRtStFtrstIsTargetPosAlready_Val_read)
  MdXXSecRwRtStFtrstIsTargetPosZone_Val_read/1 -> Subsystem/28(MdXXSecRwRtStFtrstIsTargetPosZone_Val_read)
  MdXXSecRwRtStFwdBkwdIsTargetPosAlready_Val_read/1 -> Subsystem/29(MdXXSecRwRtStFwdBkwdIsTargetPosAlready_Val_read)
  MdXXSecRwRtStFwdBkwdIsTargetPosZone_Val_read/1 -> Subsystem/30(MdXXSecRwRtStFwdBkwdIsTargetPosZone_Val_read)
  MdXXSecRwRtStHdrstFwdBkwdIsTargetPosAlready_Val_read/1 -> Subsystem/31(MdXXSecRwRtStHdrstFwdBkwdIsTargetPosAlready_Val_read)
  MdXXSecRwRtStHdrstFwdBkwdIsTargetPosZone_Val_read/1 -> Subsystem/32(MdXXSecRwRtStHdrstFwdBkwdIsTargetPosZone_Val_read)
  MdXXSecRwRtStHdrstUpwdDnwdIsTargetPosAlready_Val_read/1 -> Subsystem/33(MdXXSecRwRtStHdrstUpwdDnwdIsTargetPosAlready_Val_read)
  MdXXSecRwRtStHdrstUpwdDnwdIsTargetPosZone_Val_read/1 -> Subsystem/34(MdXXSecRwRtStHdrstUpwdDnwdIsTargetPosZone_Val_read)
  MdXXSecRwRtStLgrstInwdOtwdIsTargetPosAlready_Val_read/1 -> Subsystem/35(MdXXSecRwRtStLgrstInwdOtwdIsTargetPosAlready_Val_read)
  MdXXSecRwRtStLgrstInwdOtwdIsTargetPosZone_Val_read/1 -> Subsystem/36(MdXXSecRwRtStLgrstInwdOtwdIsTargetPosZone_Val_read)
  MdXXSecRwRtStLgrstUpwdDnwdIsTargetPosAlready_Val_read/1 -> Subsystem/37(MdXXSecRwRtStLgrstUpwdDnwdIsTargetPosAlready_Val_read)
  MdXXSecRwRtStLgrstUpwdDnwdIsTargetPosZone_Val_read/1 -> Subsystem/38(MdXXSecRwRtStLgrstUpwdDnwdIsTargetPosZone_Val_read)
  MdXXSecRwRtStLtwdRtwdIsTargetPosAlready_Val_read/1 -> Subsystem/39(MdXXSecRwRtStLtwdRtwdIsTargetPosAlready_Val_read)
  MdXXSecRwRtStLtwdRtwdIsTargetPosZone_Val_read/1 -> Subsystem/40(MdXXSecRwRtStLtwdRtwdIsTargetPosZone_Val_read)
  MdXXThdRwLtStBkReclnIsTargetPosAlready_Val_read/1 -> Subsystem/41(MdXXThdRwLtStBkReclnIsTargetPosAlready_Val_read)
  MdXXThdRwLtStBkReclnIsTargetPosZone_Val_read/1 -> Subsystem/42(MdXXThdRwLtStBkReclnIsTargetPosZone_Val_read)
  MdXXThdRwLtStCshnFldIsTargetPosAlready_Val_read/1 -> Subsystem/43(MdXXThdRwLtStCshnFldIsTargetPosAlready_Val_read)
  MdXXThdRwLtStCshnFldIsTargetPosZone_Val_read/1 -> Subsystem/44(MdXXThdRwLtStCshnFldIsTargetPosZone_Val_read)
  MdXXThdRwLtStFwdBkwdIsTargetPosAlready_Val_read/1 -> Subsystem/45(MdXXThdRwLtStFwdBkwdIsTargetPosAlready_Val_read)
  MdXXThdRwLtStFwdBkwdIsTargetPosZone_Val_read/1 -> Subsystem/46(MdXXThdRwLtStFwdBkwdIsTargetPosZone_Val_read)
  MdXXThdRwRtStBkReclnIsTargetPosAlready_Val_read/1 -> Subsystem/47(MdXXThdRwRtStBkReclnIsTargetPosAlready_Val_read)
  MdXXThdRwRtStBkReclnIsTargetPosZone_Val_read/1 -> Subsystem/48(MdXXThdRwRtStBkReclnIsTargetPosZone_Val_read)
  MdXXThdRwRtStCshnFldIsTargetPosAlready_Val_read/1 -> Subsystem/49(MdXXThdRwRtStCshnFldIsTargetPosAlready_Val_read)
  MdXXThdRwRtStCshnFldIsTargetPosZone_Val_read/1 -> Subsystem/50(MdXXThdRwRtStCshnFldIsTargetPosZone_Val_read)
  MdXXThdRwRtStFwdBkwdIsTargetPosAlready_Val_read/1 -> Subsystem/51(MdXXThdRwRtStFwdBkwdIsTargetPosAlready_Val_read)
  MdXXThdRwRtStFwdBkwdIsTargetPosZone_Val_read/1 -> Subsystem/52(MdXXThdRwRtStFwdBkwdIsTargetPosZone_Val_read)
  Subsystem/1(MdXXIsTargetPosAlready_Val_write) -> MdXXIsTargetPosAlready_Val_write/1
  Subsystem/2(MdXXIsTargetPosZone_Val_write) -> MdXXIsTargetPosZone_Val_write/1
  MdXXSecRwLtStZeroIsTargetPosZone_Val_read/1 -> Subsystem/54(MdXXSecRwLtStZeroIsTargetPosZone_Val_read)
  MdXXSecRwRtStZeroIsTargetPosAlready_Val_read/1 -> Subsystem/55(MdXXSecRwRtStZeroIsTargetPosAlready_Val_read)
  MdXXSecRwRtStZeroIsTargetPosZone_Val_read/1 -> Subsystem/56(MdXXSecRwRtStZeroIsTargetPosZone_Val_read)
  MdXXSecRwLtStZeroIsTargetPosAlready_Val_read/1 -> Subsystem/53(MdXXSecRwLtStZeroIsTargetPosAlready_Val_read)
  MdXXPassStBkReclnIsTargetPosAlready_Val_read/1 -> Subsystem/57(MdXXPassStBkReclnIsTargetPosAlready_Val_read)
  MdXXPassStBkReclnIsTargetPosZone_Val_read/1 -> Subsystem/58(MdXXPassStBkReclnIsTargetPosZone_Val_read)
  MdXXPassStCshnFldIsTargetPosAlready_Val_read/1 -> Subsystem/59(MdXXPassStCshnFldIsTargetPosAlready_Val_read)
  MdXXPassStCshnFldIsTargetPosZone_Val_read/1 -> Subsystem/60(MdXXPassStCshnFldIsTargetPosZone_Val_read)
  MdXXPassStFwdBkwdIsTargetPosAlready_Val_read/1 -> Subsystem/61(MdXXPassStFwdBkwdIsTargetPosAlready_Val_read)
  MdXXPassStFwdBkwdIsTargetPosZone_Val_read/1 -> Subsystem/62(MdXXPassStFwdBkwdIsTargetPosZone_Val_read)

== system MdXXIsPosChk/MdXXIsPosChk_Init ==
  Event Listener : EventListener  EventName=reset
